simulink model "lab1c"  (R2023a)
settings: Solver=VariableStepAuto  StartTime=0.0  StopTime=10.0  RelTol=1e-3
settings Model: Creator=CSE-LAB2-64  LastModifiedBy=CSE-LAB2-64

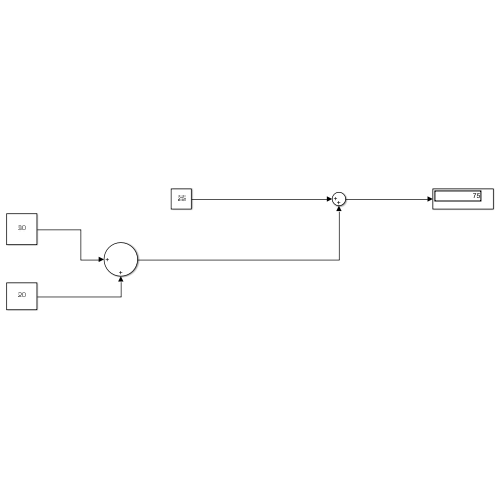
[thumbnail: Simulink's stored preview of the top-level diagram]
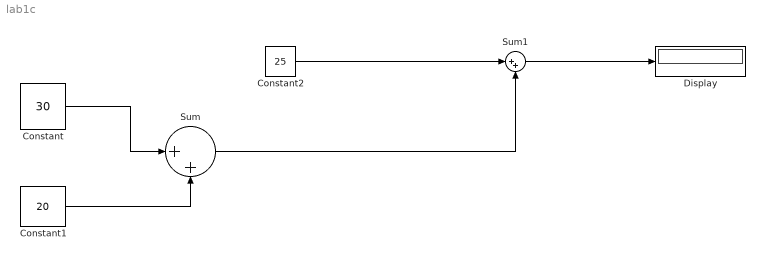
== system lab1c ==
  Constant : Constant  Value=30
  Constant1 : Constant  Value=20
  Constant2 : Constant  Value=25
  Display : Display
  Sum : Sum  Inputs=|++
  Sum1 : Sum  Inputs=|++
  wires:
  Constant/1 -> Sum/1
  Constant1/1 -> Sum/2
  Sum/1 -> Sum1/2
  Constant2/1 -> Sum1/1
  Sum1/1 -> Display/1
